simulink model "biped_robot_forward_model"  (R2017a)
settings: Solver=FixedStepAuto  StartTime=0.0  StopTime=10  FixedStep=0.000025  MaxStep=1e-4  RelTol=1e-3
model workspace (MAT data in the model file):
  Sig = Simulink.Signal
  Sig.DataType = 'auto'
  Sig.Dimensions = -1
  Sig.DimensionsMode = 'auto'
  Sig.Complexity = 'auto'
  Sig.SampleTime = -1
  Sig.SamplingMode = 'auto'
  angles.time = []
  angles.signals.dimensions = 12
  angles.signals.values = [0 0 0 0 0 0 0 0 0 0 0 0 ... (24000 elements, 2000x12)]
  body.height = 0.14
  body.width = 0.15
  body.depth = 0.08
  body_mass = 1.5508
  collider_radius = 0.005
  dh = [0.025  -1.57079632679  0  1.57079632679; 0  1.57079632679  0  -1.57079632679; 0  0  0.089  0; 0  0  0.0825  0; 0  0  0  1.57079632679; 0  0  0.037  0]
  gravity = -9.81
  ground.depth = 0.01
  ground.width = 1
  ground.length = 5
  hip_width = 0.08
  init_body_height = 0.259
  kd = 0
  ki = 0
  kp = 100
  link_masses = [0.04589; 0.16336; 0.15143; 0.06792]
  q0_left = [0; -0.044595249101; 1.01873631358; -1.40418241322; 0.385446099643; 0.044595249101]
  q0_right = [0; -0.204334326062; 0.671750415328; -1.49726195766; 0.825511542331; 0.204334326062]
undefined symbols (not defined in the file): X, Y, Z
libraries: sm_lib x15, biped_robot_library x14, nesl_utility x11, neural x1, simulink x1
settings Model: Creator=Lukas  LastModifiedBy=Lukas

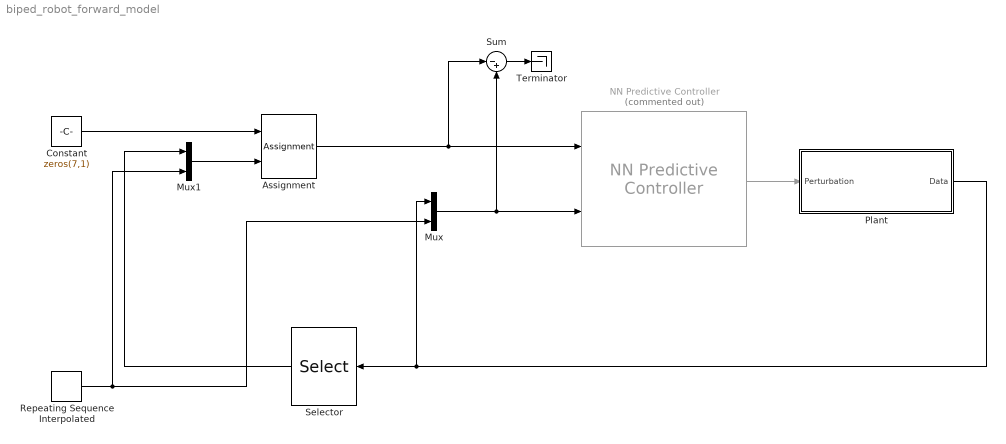
== system biped_robot_forward_model ==
  Assignment : Assignment  DiagnosticForDimensions=Warning  IndexOptions=Index vector (dialog)  Indices=[4 7]  OutputSizes=1
  Constant : Constant  Value=zeros(7,1)
  Mux : Mux  Inputs=[6 1]
  Mux1 : Mux  Inputs=2
  NN Predictive Controller : neural/Control Systems/NN Predictive Controller  Commented=on  epochs=[]  minp=[]  maxp=[]  mint=[]  maxt=[]  Normalize=[]  IW=[]  LW1_2=[]  LW2_1=[]  B1=[]  B2=[]  max_i_int=[]  min_i_int=[]  limit_output=[]  max_output=[]  min_output=[]  Use_Previous_Weights=[]  N2=[]  Nu=[]  Ts=[]  rho=[]  alpha=[]  csrchfun=csrchbac  maxiter=[]  S1=[]  Ni=[]  Nj=[]  sim_file=0  trainfun=trainlm  Use_validation=[]  Use_Testing=[]  max_i=[]  min_i=[]  sam_training=[]
      settings: SourceProductName=Neural Network Toolbox  SourceProductBaseCode=NN
  Plant : Subsystem  TreatAsAtomicUnit=on  VariantControl=Variant1
  Repeating Sequence Interpolated : simulink/Sources/Repeating Sequence Interpolated  OutValues=0.01*(0:200)  TimeValues=0.01*(0:200)  LookUpMeth=Interpolation-Use End Values  tsamp=-1  OutMin=[]  OutMax=[]  OutDataTypeStr=double  OutputDataTypeScalingMode=double  OutDataType=fixdt(0,8)  OutScaling=2^-10
  Selector : Selector  InputPortWidth=6  IndexOptions=Index vector (dialog)  Indices=4  OutputSizes=1
  Sum : Sum  Inputs=|-+
  Terminator : Terminator
  wires:
  Constant/1 -> Assignment/1
  Mux/1 -> Sum/2, NN Predictive Controller/2
  Repeating Sequence Interpolated/1 -> Mux1/2, Mux/2
  Selector/1 -> Mux1/1
  Mux1/1 -> Assignment/2
  Assignment/1 -> Sum/1, NN Predictive Controller/1
  Sum/1 -> Terminator/1
  NN Predictive Controller/1 -> Plant/1(Perturbation)
  Plant/1(Data) -> Mux/1, Selector/1

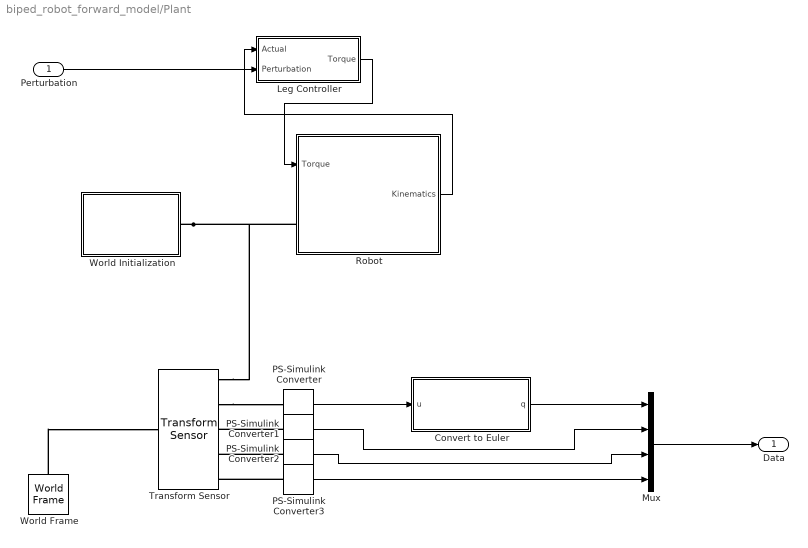
== system biped_robot_forward_model/Plant ==
  Perturbation : Inport
  Convert to Euler : MATLAB Function  TreatAsAtomicUnit=on
  Leg Controller : Subsystem
  Mux : Mux  Inputs=[3 1 1 1]
  PS-Simulink Converter{,1..3} (4 alike) : nesl_utility/PS-Simulink Converter  PhysicalDomain=network_engine_domain  SubClassName=ps_output  LeftPortType=input  RightPortType=output  PseudoPeriodic=off  Frequencies=[]  Unit=1  AffineConversion=off
  Robot : Subsystem
  Transform Sensor : sm_lib/Frames and Transforms/Transform Sensor  MeasurementFrame=World  SenseAngle=off  SenseAxis=off  SenseAngle1=off  SenseAngle2=off  SenseAngle3=off  SenseQ=on  SenseR=off  SenseOmegaX=off  SenseOmegaY=off  SenseOmegaZ=off  SenseOmega1=off  SenseOmega2=off  SenseOmega3=off  SenseQDot=off  SenseRDot=off  SenseAlphaX=off  SenseAlphaY=off  SenseAlphaZ=off  SenseAlpha1=off  SenseAlpha2=off  SenseAlpha3=off  SenseQDDot=off  SenseRDDot=off  SenseX=off  SenseY=off  SenseZ=off  SenseRad=off  SenseAzim=off  SenseDist=off  SenseInc=off  SenseXDot=off  SenseYDot=off  SenseZDot=off  SenseRadDot=off  SenseAzimDot=off  SenseDistDot=off  SenseIncDot=off  SenseXDDot=on  SenseYDDot=on  SenseZDDot=on  SenseRadDDot=off  SenseAzimDDot=off  SenseDistDDot=off  SenseIncDDot=off
  World Frame : sm_lib/Frames and Transforms/World Frame
  World Initialization : Subsystem
  Data : Outport
  wires:
  PS-Simulink Converter/1 -> Convert to Euler/1(u)
  Leg Controller/1(Torque) -> Robot/1(Torque)
  Robot/1(Kinematics) -> Leg Controller/1(Actual)
  PS-Simulink Converter2/1 -> Mux/3
  Mux/1 -> Data/1
  PS-Simulink Converter1/1 -> Mux/2
  PS-Simulink Converter3/1 -> Mux/4
  Perturbation/1 -> Leg Controller/2(Perturbation)
  Convert to Euler/1(q) -> Mux/1
  connections:
  PS-Simulink Converter2/LConn1 -- Transform Sensor/RConn4
  PS-Simulink Converter1/LConn1 -- Transform Sensor/RConn3
  PS-Simulink Converter3/LConn1 -- Transform Sensor/RConn5
  World Frame/RConn1 -- Transform Sensor/LConn1
  World Initialization/RConn1 -- Robot/LConn1 -- Transform Sensor/RConn1
  Transform Sensor/RConn2 -- PS-Simulink Converter/LConn1

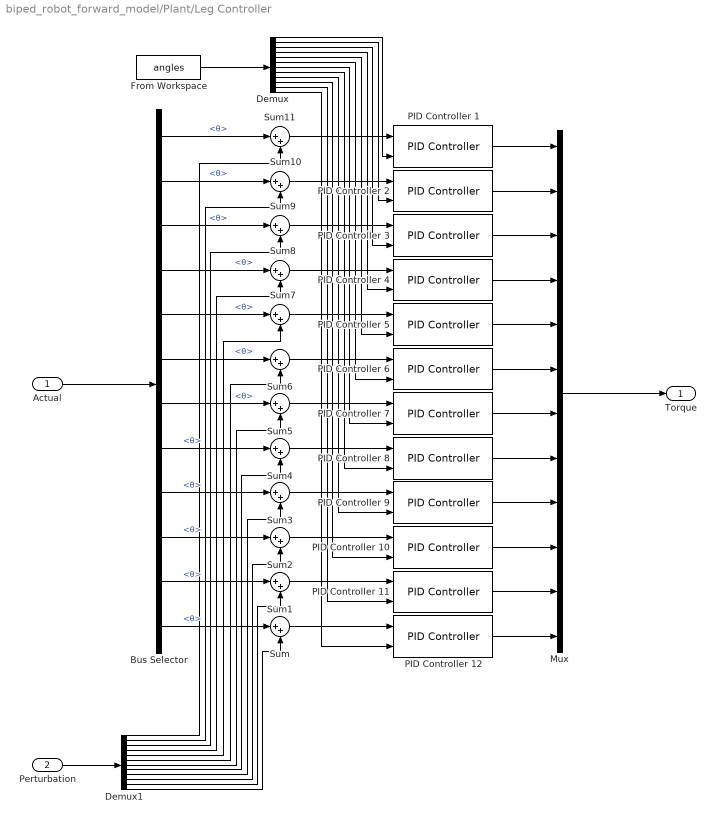
== system biped_robot_forward_model/Plant/Leg Controller ==
  Actual : Inport
  Perturbation : Inport  Port=2
  Bus Selector : BusSelector  OutputSignals=Left Leg.Hip 1.θ,Left Leg.Hip 2.θ,Left Leg.Hip 3.θ,Left Leg.Knee.θ,Left Leg.Ankle 1.θ,Left Leg.Ankle 2.θ,Right Leg.Hip 1.θ,Right Leg.Hip 2.θ,Right Leg.Hip 3.θ,Right Leg.Knee.θ,Right Leg.Ankle 1.θ,Right Leg.Ankle 2.θ
  Demux : Demux  Outputs=12
  Demux1 : Demux  Outputs=12
  From Workspace : FromWorkspace  VariableName=angles  SampleTime=0.001  Interpolate=off  OutputAfterFinalValue=Cyclic repetition
  Mux : Mux  Inputs=12
  PID Controller {1..12} (12 alike) : biped_robot_library/PID Controller  seed=23300  kp=kp  ki=kd  kd=ki
  Sum{,1..11} (12 alike) : Sum  Inputs=|++
  Torque : Outport
  wires:
  Actual/1 -> Bus Selector/1
  PID Controller 12/1 -> Mux/12
  PID Controller 1/1 -> Mux/1
  PID Controller 2/1 -> Mux/2
  PID Controller 3/1 -> Mux/3
  PID Controller 4/1 -> Mux/4
  PID Controller 5/1 -> Mux/5
  PID Controller 6/1 -> Mux/6
  PID Controller 7/1 -> Mux/7
  PID Controller 8/1 -> Mux/8
  PID Controller 9/1 -> Mux/9
  PID Controller 10/1 -> Mux/10
  PID Controller 11/1 -> Mux/11
  Demux/1 -> PID Controller 1/2
  Demux/2 -> PID Controller 2/2
  Demux/3 -> PID Controller 3/2
  Demux/4 -> PID Controller 4/2
  Demux/5 -> PID Controller 5/2
  Demux/6 -> PID Controller 6/2
  Demux/7 -> PID Controller 7/2
  Demux/8 -> PID Controller 8/2
  Demux/9 -> PID Controller 9/2
  Demux/10 -> PID Controller 10/2
  Demux/11 -> PID Controller 11/2
  Demux/12 -> PID Controller 12/2
  Mux/1 -> Torque/1
  From Workspace/1 -> Demux/1
  Sum/1 -> PID Controller 12/1
  Bus Selector/12 -> Sum/1  "<θ>"
  Bus Selector/11 -> Sum1/1  "<θ>"
  Sum1/1 -> PID Controller 11/1
  Sum2/1 -> PID Controller 10/1
  Bus Selector/10 -> Sum2/1  "<θ>"
  Sum3/1 -> PID Controller 9/1
  Bus Selector/9 -> Sum3/1  "<θ>"
  Sum4/1 -> PID Controller 8/1
  Bus Selector/8 -> Sum4/1  "<θ>"
  Sum5/1 -> PID Controller 7/1
  Bus Selector/7 -> Sum5/1  "<θ>"
  Sum6/1 -> PID Controller 6/1
  Bus Selector/6 -> Sum6/1  "<θ>"
  Sum7/1 -> PID Controller 5/1
  Bus Selector/5 -> Sum7/1  "<θ>"
  Sum8/1 -> PID Controller 4/1
  Bus Selector/4 -> Sum8/1  "<θ>"
  Sum9/1 -> PID Controller 3/1
  Bus Selector/3 -> Sum9/1  "<θ>"
  Sum10/1 -> PID Controller 2/1
  Bus Selector/2 -> Sum10/1  "<θ>"
  Sum11/1 -> PID Controller 1/1
  Bus Selector/1 -> Sum11/1  "<θ>"
  Demux1/1 -> Sum11/2
  Demux1/2 -> Sum10/2
  Demux1/3 -> Sum9/2
  Demux1/4 -> Sum8/2
  Demux1/5 -> Sum7/2
  Demux1/6 -> Sum6/2
  Demux1/7 -> Sum5/2
  Demux1/8 -> Sum4/2
  Demux1/9 -> Sum3/2
  Demux1/10 -> Sum2/2
  Demux1/11 -> Sum1/2
  Demux1/12 -> Sum/2
  Perturbation/1 -> Demux1/1

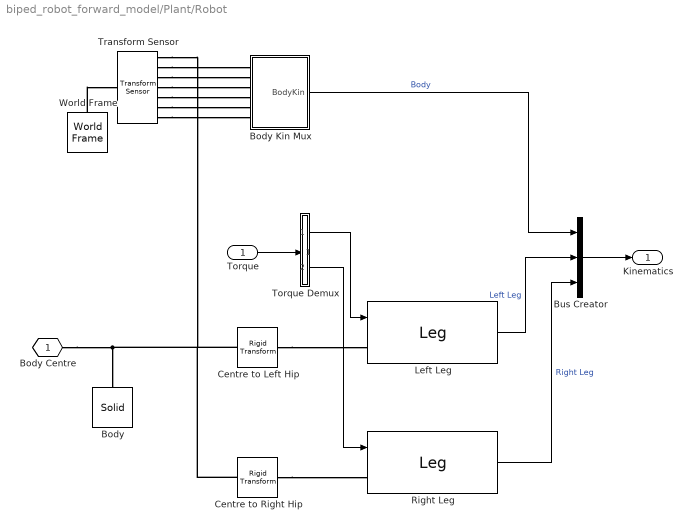
== system biped_robot_forward_model/Plant/Robot ==
  Torque : Inport
  Body : sm_lib/Body Elements/Solid  InertiaType=CalculateFromGeometry  Mass=body_mass  MassUnits=kg  CenterOfMass=[0 0 0]  CenterOfMassUnits=m  MomentsOfInertia=[1 1 1]  MomentsOfInertiaUnits=kg*m^2  ProductsOfInertia=[0 0 0]  ProductsOfInertiaUnits=kg*m^2  DensityBased=off  Density=1000  DensityUnits=kg/(m^3)  DoExposeReferenceFrame=on  SerializedFrames=<Frames/>  GraphicType=FromGeometry  MarkerShape=Sphere  MarkerSize=10  MarkerSizeUnits=m  GraphicVisPropType=SimpleVisualProperties  GraphicDiffuseColor=[0.5 0.5 0.5]  GraphicSpecularColor=[0.5 0.5 0.5 1.0]  GraphicAmbientColor=[0.15 0.15 0.15 1.0]  GraphicEmissiveColor=[0.0 0.0 0.0 1.0]  GraphicShininess=75  GraphicOpacity=1.0  GeometryShape=Brick  RectangleSize=[1 1]  RectangleSizeUnits=m  BrickDimensions=[body.depth body.width body.height]  BrickDimensionUnits=m  CylinderRadius=1  CylinderRadiusUnits=m  CylinderLength=1  CylinderLengthUnits=m  SphereRadius=1  SphereRadiusUnits=m  EllipsoidRadii=[1 1 1]  EllipsoidRadiiUnits=m  ExtrusionCrossSection=[1 1; -1 1; -1 -1; 1 -1]  ExtrusionCrossSectionUnits=m  ExtrusionLength=1  ExtrusionLengthUnits=m  PolygonNumSides=3  PolygonOuterRadius=1  PolygonOuterRadiusUnits=m  ExtGeomFileType=STEP  ExtGeomFileUnits=m  RevolutionCrossSection=[1 1; 1 -1; 2 -1; 2 1]  RevolutionCrossSectionUnits=m  RevolutionExtent=Full  RevolutionAngle=180  RevolutionAngleUnits=deg
  Body Kin Mux : Subsystem
  Bus Creator : BusCreator  Inputs=3
  Centre to Left Hip : sm_lib/Frames and Transforms/Rigid Transform  TranslationMethod=Cartesian  TranslationStandardOffset=0  TranslationLengthUnit=m  TranslationStandardAxis=+Z  TranslationCartesianOffset=[0 hip_width/2 -body.height/2]  TranslationROffset=0  TranslationROffsetUnits=m  TranslationZOffset=0  TranslationZOffsetUnits=m  TranslationThetaOffset=0  TranslationThetaOffsetUnits=deg  RotationMethod=AlignedAxes  RotationAngleUnits=deg  RotationStandardAxis=+Z  RotationAngle=0.0  RotationArbitraryAxis=[0 0 1]  FollAlignAxisA=+Z  BaseAlignAxisA=-Z  FollAlignAxisB=+X  BaseAlignAxisB=+X  RotationSequenceAxes=FollowerAxes  RotationSequence=XYX  RotationSequenceAngles=[0 0 0]  RotationSequenceAnglesUnits=deg  RotationMatrix=[1 0 0; 0 1 0; 0 0 1]
  Centre to Right Hip : sm_lib/Frames and Transforms/Rigid Transform  TranslationMethod=Cartesian  TranslationStandardOffset=0  TranslationLengthUnit=m  TranslationStandardAxis=+Z  TranslationCartesianOffset=[0 -hip_width/2 -body.height/2]  TranslationROffset=0  TranslationROffsetUnits=m  TranslationZOffset=0  TranslationZOffsetUnits=m  TranslationThetaOffset=0  TranslationThetaOffsetUnits=deg  RotationMethod=AlignedAxes  RotationAngleUnits=deg  RotationStandardAxis=+Z  RotationAngle=0.0  RotationArbitraryAxis=[0 0 1]  FollAlignAxisA=+Z  BaseAlignAxisA=-Z  FollAlignAxisB=+X  BaseAlignAxisB=+X  RotationSequenceAxes=FollowerAxes  RotationSequence=XYX  RotationSequenceAngles=[0 0 0]  RotationSequenceAnglesUnits=deg  RotationMatrix=[1 0 0; 0 1 0; 0 0 1]
  Left Leg : biped_robot_library/Leg  dh_mat=dh  q0=q0_left  lw=0.02
  Right Leg : biped_robot_library/Leg  dh_mat=dh  q0=q0_right  lw=0.02
  Torque Demux : Subsystem
  Transform Sensor : sm_lib/Frames and Transforms/Transform Sensor  MeasurementFrame=Follower  SenseAngle=off  SenseAxis=off  SenseAngle1=off  SenseAngle2=off  SenseAngle3=off  SenseQ=off  SenseR=off  SenseOmegaX=off  SenseOmegaY=off  SenseOmegaZ=off  SenseOmega1=off  SenseOmega2=off  SenseOmega3=off  SenseQDot=off  SenseRDot=off  SenseAlphaX=off  SenseAlphaY=off  SenseAlphaZ=off  SenseAlpha1=off  SenseAlpha2=off  SenseAlpha3=off  SenseQDDot=off  SenseRDDot=off  SenseX=on  SenseY=on  SenseZ=on  SenseRad=off  SenseAzim=off  SenseDist=off  SenseInc=off  SenseXDot=off  SenseYDot=off  SenseZDot=off  SenseRadDot=off  SenseAzimDot=off  SenseDistDot=off  SenseIncDot=off  SenseXDDot=on  SenseYDDot=on  SenseZDDot=on  SenseRadDDot=off  SenseAzimDDot=off  SenseDistDDot=off  SenseIncDDot=off
  World Frame : sm_lib/Frames and Transforms/World Frame
  Body Centre : PMIOPort  Tag=PMCPort  Port=1  Side=Left
  Kinematics : Outport
  wires:
  Bus Creator/1 -> Kinematics/1
  Left Leg/1 -> Bus Creator/2  "Left Leg"
  Body Kin Mux/1(BodyKin) -> Bus Creator/1  "Body"
  Right Leg/1 -> Bus Creator/3  "Right Leg"
  Torque/1 -> Torque Demux/1(Torque)
  Torque Demux/1(Left Leg Torques) -> Left Leg/1
  Torque Demux/2(Right Leg Torques) -> Right Leg/1
  connections:
  Body Centre/RConn1 -- Centre to Left Hip/LConn1 -- Transform Sensor/RConn1 -- Centre to Right Hip/LConn1 -- Body/RConn1
  World Frame/RConn1 -- Transform Sensor/LConn1
  Transform Sensor/RConn2 -- Body Kin Mux/LConn1
  Transform Sensor/RConn3 -- Body Kin Mux/LConn2
  Transform Sensor/RConn4 -- Body Kin Mux/LConn3
  Centre to Left Hip/RConn1 -- Left Leg/LConn1
  Centre to Right Hip/RConn1 -- Right Leg/LConn1
  Transform Sensor/RConn5 -- Body Kin Mux/LConn4
  Transform Sensor/RConn6 -- Body Kin Mux/LConn5
  Transform Sensor/RConn7 -- Body Kin Mux/LConn6

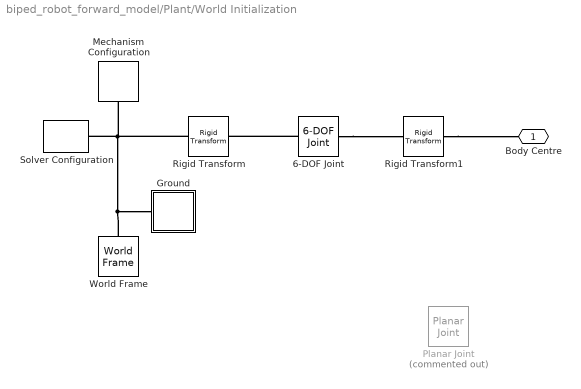
== system biped_robot_forward_model/Plant/World Initialization ==
  6-DOF Joint : sm_lib/Joints/6-DOF Joint  SenseConstraintForce=off  SenseConstraintForceX=off  SenseConstraintForceY=off  SenseConstraintForceZ=off  SenseConstraintTorque=off  SenseConstraintTorqueX=off  SenseConstraintTorqueY=off  SenseConstraintTorqueZ=off  SenseTotalForce=off  SenseTotalForceX=off  SenseTotalForceY=off  SenseTotalForceZ=off  SenseTotalTorque=off  SenseTotalTorqueX=off  SenseTotalTorqueY=off  SenseTotalTorqueZ=off  CompositeWrenchDir=FollowerOnBase  CompositeWrenchFrame=BaseFrame  PxEquilibriumPosition=0  PxEquilibriumPositionUnits=m  PxSpringStiffness=0  PxSpringStiffnessUnits=N/m  PxDampingCoefficient=0  PxDampingCoefficientUnits=N/(m/s)  PxTorqueActuationMode=NoTorque  PxMotionActuationMode=ComputedMotion  PxSensePosition=off  PxSenseVelocity=off  PxSenseAcceleration=off  PxSenseTorqueForce=off  PxPositionTargetSpecify=on  PxPositionTargetPriority=High  PxPositionTargetValue=init_body_height  PxPositionTargetValueUnits=m  PxVelocityTargetSpecify=off  PxVelocityTargetPriority=High  PxVelocityTargetValue=0  PxVelocityTargetValueUnits=m/s  PyEquilibriumPosition=0  PyEquilibriumPositionUnits=m  PySpringStiffness=0  PySpringStiffnessUnits=N/m  PyDampingCoefficient=0  PyDampingCoefficientUnits=N/(m/s)  PyTorqueActuationMode=NoTorque  PyMotionActuationMode=ComputedMotion  PySensePosition=off  PySenseVelocity=off  PySenseAcceleration=off  PySenseTorqueForce=off  PyPositionTargetSpecify=off  PyPositionTargetPriority=High  PyPositionTargetValue=0  PyPositionTargetValueUnits=m  PyVelocityTargetSpecify=off  PyVelocityTargetPriority=High  PyVelocityTargetValue=0  PyVelocityTargetValueUnits=m/s  PzEquilibriumPosition=0  PzEquilibriumPositionUnits=m  PzSpringStiffness=0  PzSpringStiffnessUnits=N/m  PzDampingCoefficient=0  PzDampingCoefficientUnits=N/(m/s)  PzTorqueActuationMode=NoTorque  PzMotionActuationMode=ComputedMotion  PzSensePosition=off  PzSenseVelocity=off  PzSenseAcceleration=off  PzSenseTorqueForce=off  PzPositionTargetSpecify=off  PzPositionTargetPriority=High  PzPositionTargetValue=0  PzPositionTargetValueUnits=m  PzVelocityTargetSpecify=off  PzVelocityTargetPriority=High  PzVelocityTargetValue=0  PzVelocityTargetValueUnits=m/s  SphDefPosRotationMethod=None  SphDefPosRotationAngleUnits=deg  SphDefPosRotationStandardAxis=+Z  SphDefPosRotationAngle=0.0  SphDefPosRotationArbitraryAxis=[0 0 1]  SphDefPosFollAlignAxisA=+X  SphDefPosBaseAlignAxisA=+Y  SphDefPosFollAlignAxisB=+Y  SphDefPosBaseAlignAxisB=+Z  SphDefPosRotationSequenceAxes=FollowerAxes  SphDefPosRotationSequence=XYX  SphDefPosRotationSequenceAngles=[0 0 0]  SphDefPosRotationSequenceAnglesUnits=deg  SphDefPosRotationMatrix=[1 0 0; 0 1 0; 0 0 1]  SphEqPosRotationMethod=None  SphEqPosRotationAngleUnits=deg  SphEqPosRotationStandardAxis=+Z  SphEqPosRotationAngle=0.0  SphEqPosRotationArbitraryAxis=[0 0 1]  SphEqPosFollAlignAxisA=+X  SphEqPosBaseAlignAxisA=+Y  SphEqPosFollAlignAxisB=+Y  SphEqPosBaseAlignAxisB=+Z  SphEqPosRotationSequenceAxes=FollowerAxes  SphEqPosRotationSequence=XYX  SphEqPosRotationSequenceAngles=[0 0 0]  SphEqPosRotationSequenceAnglesUnits=deg  SphEqPosRotationMatrix=[1 0 0; 0 1 0; 0 0 1]  SphSpringStiffness=0  SphSpringStiffnessUnits=N*m/deg  SphDampingCoefficient=0  SphDampingCoefficientUnits=N*m/(deg/s)  SphActuateTorqueX=off  SphActuateTorqueY=off  SphActuateTorqueZ=off  SphActuateTorque=off  SphTorqueActuationMode=NoTorque  SphMotionActuationMode=ComputedMotion  SphActuationFrame=BaseFrame  SphSensePosition=off  SphSenseVelocityX=off  SphSenseVelocityY=off  SphSenseVelocityZ=off  SphSenseVelocity=off  SphSenseAccelerationX=off  SphSenseAccelerationY=off  SphSenseAccelerationZ=off  SphSenseAcceleration=off  SphSenseTorqueX=off  SphSenseTorqueY=off  SphSenseTorqueZ=off  SphSenseTorqueForce=off  SphSensingFrame=BaseFrame  SphPositionTargetRotationMethod=None  SphPositionTargetRotationAngleUnits=deg  SphPositionTargetRotationStandardAxis=+Z  SphPositionTargetRotationAngle=0.0  SphPositionTargetRotationArbitraryAxis=[0 0 1]  SphPositionTargetFollAlignAxisA=+X  SphPositionTargetBaseAlignAxisA=+Y  SphPositionTargetFollAlignAxisB=+Y  SphPositionTargetBaseAlignAxisB=+Z  SphPositionTargetRotationSequenceAxes=FollowerAxes  SphPositionTargetRotationSequence=XYX  SphPositionTargetRotationSequenceAngles=[0 0 0]  SphPositionTargetRotationSequenceAnglesUnits=deg  SphPositionTargetRotationMatrix=[1 0 0; 0 1 0; 0 0 1]  SphPositionTargetSpecify=off  SphPositionTargetPriority=High  SphVelocityTargetValue=[0 0 0]  SphVelocityTargetValueUnits=deg/s  SphVelocityTargetSpecify=off  SphVelocityTargetPriority=High  SphVelocityTargetInFollowerFrame=on
  Ground : Subsystem
  Mechanism Configuration : sm_lib/Utilities/Mechanism Configuration  UniformGravity=Constant  GravityVector=[0 0 gravity]  GravityUnits=m/s^2  LinearizationDelta=0.001
  Planar Joint : sm_lib/Joints/Planar Joint  Commented=on  SenseConstraintForce=off  SenseConstraintForceX=off  SenseConstraintForceY=off  SenseConstraintForceZ=off  SenseConstraintTorque=off  SenseConstraintTorqueX=off  SenseConstraintTorqueY=off  SenseConstraintTorqueZ=off  SenseTotalForce=off  SenseTotalForceX=off  SenseTotalForceY=off  SenseTotalForceZ=off  SenseTotalTorque=off  SenseTotalTorqueX=off  SenseTotalTorqueY=off  SenseTotalTorqueZ=off  CompositeWrenchDir=FollowerOnBase  CompositeWrenchFrame=BaseFrame  PxEquilibriumPosition=0  PxEquilibriumPositionUnits=m  PxSpringStiffness=0  PxSpringStiffnessUnits=N/m  PxDampingCoefficient=0  PxDampingCoefficientUnits=N/(m/s)  PxTorqueActuationMode=NoTorque  PxMotionActuationMode=ComputedMotion  PxSensePosition=off  PxSenseVelocity=off  PxSenseAcceleration=off  PxSenseTorqueForce=off  PxPositionTargetSpecify=on  PxPositionTargetPriority=High  PxPositionTargetValue=init_body_height  PxPositionTargetValueUnits=m  PxVelocityTargetSpecify=off  PxVelocityTargetPriority=High  PxVelocityTargetValue=0  PxVelocityTargetValueUnits=m/s  PyEquilibriumPosition=0  PyEquilibriumPositionUnits=m  PySpringStiffness=0  PySpringStiffnessUnits=N/m  PyDampingCoefficient=0  PyDampingCoefficientUnits=N/(m/s)  PyTorqueActuationMode=NoTorque  PyMotionActuationMode=ComputedMotion  PySensePosition=off  PySenseVelocity=off  PySenseAcceleration=off  PySenseTorqueForce=off  PyPositionTargetSpecify=off  PyPositionTargetPriority=High  PyPositionTargetValue=0  PyPositionTargetValueUnits=m  PyVelocityTargetSpecify=off  PyVelocityTargetPriority=High  PyVelocityTargetValue=0  PyVelocityTargetValueUnits=m/s  RzEquilibriumPosition=0  RzEquilibriumPositionUnits=deg  RzSpringStiffness=0  RzSpringStiffnessUnits=N*m/deg  RzDampingCoefficient=0  RzDampingCoefficientUnits=N*m/(deg/s)  RzTorqueActuationMode=NoTorque  RzMotionActuationMode=ComputedMotion  RzSensePosition=off  RzSenseVelocity=off  RzSenseAcceleration=off  RzSenseTorqueForce=off  RzPositionTargetSpecify=off  RzPositionTargetPriority=High  RzPositionTargetValue=0  RzPositionTargetValueUnits=deg  RzVelocityTargetSpecify=off  RzVelocityTargetPriority=High  RzVelocityTargetValue=0  RzVelocityTargetValueUnits=deg/s
  Rigid Transform : sm_lib/Frames and Transforms/Rigid Transform  TranslationMethod=None  TranslationStandardOffset=0  TranslationLengthUnit=m  TranslationStandardAxis=+Z  TranslationCartesianOffset=[0 0 0]  TranslationROffset=0  TranslationROffsetUnits=m  TranslationZOffset=0  TranslationZOffsetUnits=m  TranslationThetaOffset=0  TranslationThetaOffsetUnits=deg  RotationMethod=AlignedAxes  RotationAngleUnits=deg  RotationStandardAxis=+Z  RotationAngle=0.0  RotationArbitraryAxis=[0 0 1]  FollAlignAxisA=+X  BaseAlignAxisA=+Z  FollAlignAxisB=+Z  BaseAlignAxisB=+Y  RotationSequenceAxes=FollowerAxes  RotationSequence=XYX  RotationSequenceAngles=[0 0 0]  RotationSequenceAnglesUnits=deg  RotationMatrix=[1 0 0; 0 1 0; 0 0 1]
  Rigid Transform1 : sm_lib/Frames and Transforms/Rigid Transform  TranslationMethod=StandardAxis  TranslationStandardOffset=0  TranslationLengthUnit=m  TranslationStandardAxis=+Z  TranslationCartesianOffset=[0 0 0]  TranslationROffset=0  TranslationROffsetUnits=m  TranslationZOffset=0  TranslationZOffsetUnits=m  TranslationThetaOffset=0  TranslationThetaOffsetUnits=deg  RotationMethod=AlignedAxes  RotationAngleUnits=deg  RotationStandardAxis=+Z  RotationAngle=0.0  RotationArbitraryAxis=[0 0 1]  FollAlignAxisA=+Z  BaseAlignAxisA=+X  FollAlignAxisB=+Y  BaseAlignAxisB=+Z  RotationSequenceAxes=FollowerAxes  RotationSequence=XYX  RotationSequenceAngles=[0 0 0]  RotationSequenceAnglesUnits=deg  RotationMatrix=[1 0 0; 0 1 0; 0 0 1]
  Solver Configuration : nesl_utility/Solver Configuration  PhysicalDomain=network_engine_domain  SubClassName=solver  LeftPortType=input  RightPortType=generic  Accelerate=off  Tones=[]  Harmonics=[]  SimulateNoise=off  Profile=off  UseLocalSampling=off  EnableSwitchedLinearOptims=on  FrequencyDomain=off  UseCCode=off  RelTol=0.001  AbsTol=1e-06  MinStep=1e-09  ToWorkspace=off  RevertToSquareIcSolve=off  NumHomotopyIterations=100  PhasorMode=off  PhasorModeNumHarmonics=1  OverrideAbsTol=off  DoDC=off  ResidualTolerance=1e-09  UseLocalSolver=off  LocalSolverChoice=NE_BACKWARD_EULER_ADVANCER  LocalSolverSampleTime=0.001  DoFixedCost=off  MaxNonlinIter=3  MaxModeIter=2  LinearAlgebra=Sparse  DelaysMemoryBudget=1024  AutomaticFiltering=on  FilteringTimeConstant=0.001
  World Frame : sm_lib/Frames and Transforms/World Frame
  Body Centre : PMIOPort  Port=1  Side=Right
  connections:
  6-DOF Joint/RConn1 -- Rigid Transform1/LConn1
  Rigid Transform/LConn1 -- Solver Configuration/RConn1 -- World Frame/RConn1 -- Ground/LConn1 -- Mechanism Configuration/RConn1
  Rigid Transform1/RConn1 -- Body Centre/RConn1
  6-DOF Joint/LConn1 -- Rigid Transform/RConn1

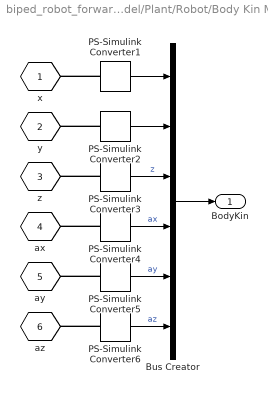
== system biped_robot_forward_model/Plant/Robot/Body Kin Mux ==
  Bus Creator : BusCreator  Inputs=6
  PS-Simulink Converter{1..6} (6 alike) : nesl_utility/PS-Simulink Converter  PhysicalDomain=network_engine_domain  SubClassName=ps_output  LeftPortType=input  RightPortType=output  PseudoPeriodic=off  Frequencies=[]  Unit=1  AffineConversion=off
  x : PMIOPort  Tag=PMCPort  Port=1  Side=Left
  y : PMIOPort  Tag=PMCPort  Port=2  Side=Left
  z : PMIOPort  Tag=PMCPort  Port=3  Side=Left
  ax : PMIOPort  Tag=PMCPort  Port=4  Side=Left
  ay : PMIOPort  Tag=PMCPort  Port=5  Side=Left
  az : PMIOPort  Tag=PMCPort  Port=6  Side=Left
  BodyKin : Outport
  wires:
  Bus Creator/1 -> BodyKin/1
  PS-Simulink Converter6/1 -> Bus Creator/6  "az"
  PS-Simulink Converter5/1 -> Bus Creator/5  "ay"
  PS-Simulink Converter4/1 -> Bus Creator/4  "ax"
  PS-Simulink Converter3/1 -> Bus Creator/3  "z"
  PS-Simulink Converter2/1 -> Bus Creator/2
  PS-Simulink Converter1/1 -> Bus Creator/1
  connections:
  PS-Simulink Converter3/LConn1 -- z/RConn1
  PS-Simulink Converter4/LConn1 -- ax/RConn1
  PS-Simulink Converter5/LConn1 -- ay/RConn1
  PS-Simulink Converter6/LConn1 -- az/RConn1
  PS-Simulink Converter1/LConn1 -- x/RConn1
  PS-Simulink Converter2/LConn1 -- y/RConn1

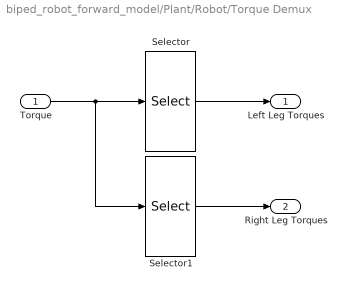
== system biped_robot_forward_model/Plant/Robot/Torque Demux ==
  Torque : Inport
  Selector : Selector  IndexMode=Zero-based  InputPortWidth=12  IndexOptions=Index vector (dialog)  Indices=0:5  OutputSizes=1
  Selector1 : Selector  IndexMode=Zero-based  InputPortWidth=12  IndexOptions=Index vector (dialog)  Indices=6:11  OutputSizes=1
  Left Leg Torques : Outport
  Right Leg Torques : Outport  Port=2
  wires:
  Selector/1 -> Left Leg Torques/1
  Selector1/1 -> Right Leg Torques/1
  Torque/1 -> Selector1/1, Selector/1

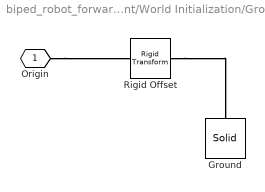
== system biped_robot_forward_model/Plant/World Initialization/Ground ==
  Ground : sm_lib/Body Elements/Solid  InertiaType=CalculateFromGeometry  Mass=1  MassUnits=kg  CenterOfMass=[0 0 0]  CenterOfMassUnits=m  MomentsOfInertia=[1 1 1]  MomentsOfInertiaUnits=kg*m^2  ProductsOfInertia=[0 0 0]  ProductsOfInertiaUnits=kg*m^2  DensityBased=on  Density=1000  DensityUnits=kg/(m^3)  DoExposeReferenceFrame=on  SerializedFrames=<Frames/>  GraphicType=FromGeometry  MarkerShape=Sphere  MarkerSize=10  MarkerSizeUnits=m  GraphicVisPropType=SimpleVisualProperties  GraphicDiffuseColor=[0.0 0.8 0.2]  GraphicSpecularColor=[0.5 0.5 0.5 1.0]  GraphicAmbientColor=[0.15 0.15 0.15 1.0]  GraphicEmissiveColor=[0.0 0.0 0.0 1.0]  GraphicShininess=75  GraphicOpacity=1.0  GeometryShape=Brick  RectangleSize=[1 1]  RectangleSizeUnits=m  BrickDimensions=[ground.length ground.width ground.depth]  BrickDimensionUnits=m  CylinderRadius=1  CylinderRadiusUnits=m  CylinderLength=1  CylinderLengthUnits=m  SphereRadius=1  SphereRadiusUnits=m  EllipsoidRadii=[1 1 1]  EllipsoidRadiiUnits=m  ExtrusionCrossSection=[1 1; -1 1; -1 -1; 1 -1]  ExtrusionCrossSectionUnits=m  ExtrusionLength=1  ExtrusionLengthUnits=m  PolygonNumSides=3  PolygonOuterRadius=1  PolygonOuterRadiusUnits=m  ExtGeomFileType=STEP  ExtGeomFileUnits=m  RevolutionCrossSection=[1 1; 1 -1; 2 -1; 2 1]  RevolutionCrossSectionUnits=m  RevolutionExtent=Full  RevolutionAngle=180  RevolutionAngleUnits=deg
  Rigid Offset : sm_lib/Frames and Transforms/Rigid Transform  TranslationMethod=StandardAxis  TranslationStandardOffset=ground.depth/2  TranslationLengthUnit=m  TranslationStandardAxis=-Z  TranslationCartesianOffset=[0 0 0]  TranslationROffset=0  TranslationROffsetUnits=m  TranslationZOffset=0  TranslationZOffsetUnits=m  TranslationThetaOffset=0  TranslationThetaOffsetUnits=deg  RotationMethod=None  RotationAngleUnits=deg  RotationStandardAxis=+Z  RotationAngle=0  RotationArbitraryAxis=[0 0 1]  FollAlignAxisA=+X  BaseAlignAxisA=+Y  FollAlignAxisB=+Y  BaseAlignAxisB=+Z  RotationSequenceAxes=FollowerAxes  RotationSequence=XYX  RotationSequenceAngles=[0 0 0]  RotationSequenceAnglesUnits=deg  RotationMatrix=[1 0 0; 0 1 0; 0 0 1]
  Origin : PMIOPort  Tag=PMCPort  Port=1  Side=Left
  connections:
  Origin/RConn1 -- Rigid Offset/LConn1
  Rigid Offset/RConn1 -- Ground/RConn1

== matlab function biped_robot_forward_model/Plant/Convert to Euler ==
  data: u input; q output
function q = convert_to_euler(u)

q = quat2eul(u');
